simulink model "untitled"  (R2014b)
settings: Solver=ode45  StartTime=0.0  StopTime=10.0  RelTol=1e-3
libraries: simulink x1
settings Model: Creator=ABDO  LastModifiedBy=ABDO

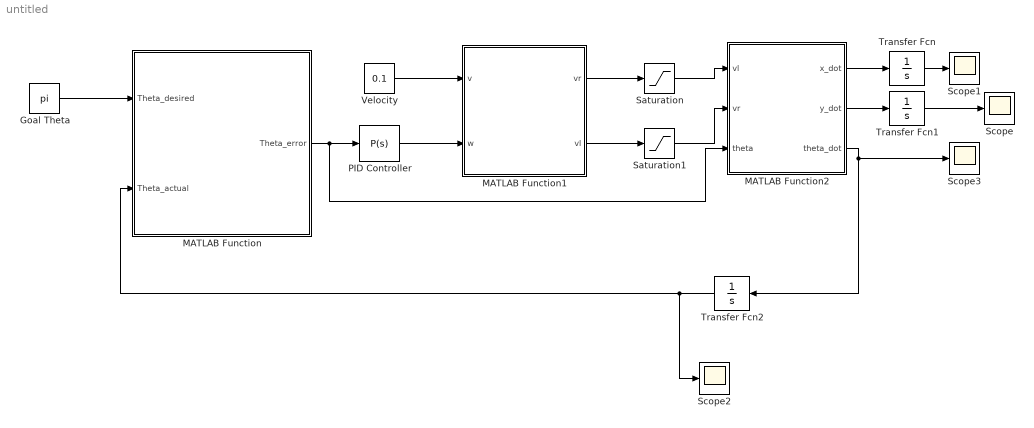
== system untitled ==
  Goal Theta : Constant  Value=pi
  MATLAB Function : MATLAB Function  TreatAsAtomicUnit=on
  MATLAB Function1 : MATLAB Function  TreatAsAtomicUnit=on
  MATLAB Function2 : MATLAB Function  TreatAsAtomicUnit=on
  PID Controller : simulink/Continuous/PID Controller  Controller=P  TimeDomain=Continuous-time  SampleTime=-1  IntegratorMethod=Forward Euler  FilterMethod=Forward Euler  Form=Parallel  P=2  I=1  D=0  N=100  InitialConditionSource=internal  InitialConditionForIntegrator=0  InitialConditionForFilter=0  ExternalReset=none  LimitOutput=off  UpperSaturationLimit=inf  LowerSaturationLimit=-inf  LinearizeAsGain=on  AntiWindupMode=none  Kb=1  TrackingMode=off  Kt=1  PParamMin=[]  PParamMax=[]  IParamMin=[]  IParamMax=[]  DParamMin=[]  DParamMax=[]  NParamMin=[]  NParamMax=[]  KbParamMin=[]  KbParamMax=[]  KtParamMin=[]  KtParamMax=[]  POutMin=[]  POutMax=[]  IOutMin=[]  IOutMax=[]  DOutMin=[]  DOutMax=[]  NOutMin=[]  NOutMax=[]  KbOutMin=[]  KbOutMax=[]  KtOutMin=[]  KtOutMax=[]  IntegratorOutMin=[]  IntegratorOutMax=[]  FilterOutMin=[]  FilterOutMax=[]  SumOutMin=[]  SumOutMax=[]  SumI1OutMin=[]  SumI1OutMax=[]  SumI2OutMin=[]  SumI2OutMax=[]  SumI3OutMin=[]  SumI3OutMax=[]  SumDOutMin=[]  SumDOutMax=[]  SaturationOutMin=[]  SaturationOutMax=[]  IntegratorContinuousStateAttributes=''  IntegratorStateMustResolveToSignalObject=off  IntegratorRTWStateStorageClass=Auto  FilterContinuousStateAttributes=''  FilterStateMustResolveToSignalObject=off  FilterRTWStateStorageClass=Auto  DifferentiatorICPrevScaledInput=0  DifferentiatorOutMin=[]  DifferentiatorOutMax=[]  UseFilter=on
  Saturation : Saturate  UpperLimit=0.41  LowerLimit=-0.41
  Saturation1 : Saturate  UpperLimit=0.41  LowerLimit=-0.41
  Scope{,1..3} (4 alike) : Scope
      Scope2 settings: SaveName=ScopeData2
      Scope3 settings: SaveName=ScopeData3
  Transfer Fcn : TransferFcn  Denominator=[1 0]
  Transfer Fcn1 : TransferFcn  Denominator=[1 0]
  Transfer Fcn2 : TransferFcn  Denominator=[1 0]
  Velocity : Constant  Value=0.1
  wires:
  Goal Theta/1 -> MATLAB Function/1(Theta_desired)
  PID Controller/1 -> MATLAB Function1/2(w)
  Velocity/1 -> MATLAB Function1/1(v)
  MATLAB Function1/1(vr) -> Saturation/1
  MATLAB Function1/2(vl) -> Saturation1/1
  Saturation/1 -> MATLAB Function2/1(vl)
  Saturation1/1 -> MATLAB Function2/2(vr)
  MATLAB Function2/1(x_dot) -> Transfer Fcn/1
  MATLAB Function2/2(y_dot) -> Transfer Fcn1/1
  MATLAB Function2/3(theta_dot) -> Scope3/1, Transfer Fcn2/1
  Transfer Fcn2/1 -> Scope2/1, MATLAB Function/2(Theta_actual)
  Transfer Fcn/1 -> Scope1/1
  Transfer Fcn1/1 -> Scope/1
  MATLAB Function/1(Theta_error) -> MATLAB Function2/3(theta), PID Controller/1

== matlab function untitled/MATLAB Function1 ==
  data: v input; vr output; w input; vl output
function [vr,vl]= fcn(v,w)
l=0.15;
vr = v+w*l/2;
vl = v-w*l/2;

== matlab function untitled/MATLAB Function ==
  data: Theta_desired input; Theta_error output; Theta_actual input
function Theta_error = Error(Theta_desired,Theta_actual)
%#codegen

Theta_error = Theta_desired-Theta_actual;

== matlab function untitled/MATLAB Function2 ==
  data: vl input; x_dot output; vr input; y_dot output; theta_dot output; theta input
function [x_dot,y_dot,theta_dot]  = fcn(vl,vr,theta)
V=(vr+vl)/2;
W=(vr-vl)/2;
x_dot=V*cos(theta);
y_dot=V*sin(theta);
theta_dot=W;
